simulink model "L0106"  (R2022b)
settings: Solver=VariableStepAuto  StartTime=0.0  StopTime=10.0  RelTol=1e-3
settings Model: Creator=Andrey  LastModifiedBy=Andrey

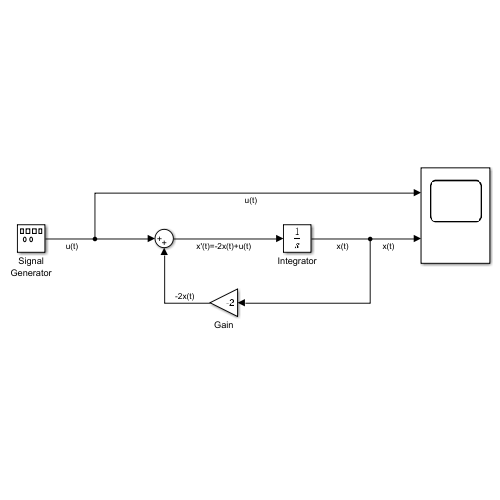
[thumbnail: Simulink's stored preview of the top-level diagram]
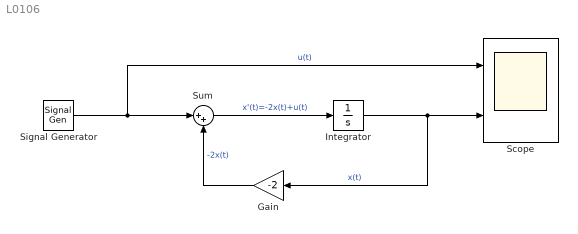
== system L0106 ==
  Gain : Gain  Gain=-2
  Integrator : Integrator
  Scope : Scope  NumInputPorts=2
  Signal Generator : SignalGenerator  WaveForm=square  Units=rad/sec
  Sum : Sum  Inputs=|++
  wires:
  Signal Generator/1 -> Scope/1, Sum/1  "u(t)"
  Sum/1 -> Integrator/1  "x'(t)=-2x(t)+u(t)"
  Integrator/1 -> Gain/1, Scope/2  "x(t)"
  Gain/1 -> Sum/2  "-2x(t)"
